simulink model "independentSISO_2023b_mdl"  (R2023b)
settings: Solver=ode4  StartTime=0  StopTime=6e6  FixedStep=0.1  RelTol=1e-3
undefined symbols (not defined in the file): f_ii, g_ii, P0
settings Model: SimulationMode=accelerator  Creator=mohammadodeh  LastModifiedBy=mohammadodeh

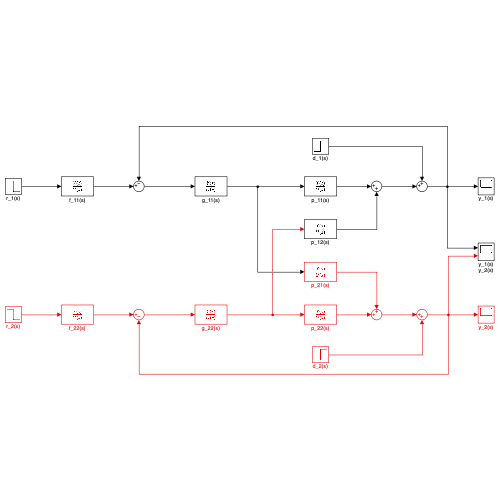
[thumbnail: Simulink's stored preview of the top-level diagram]
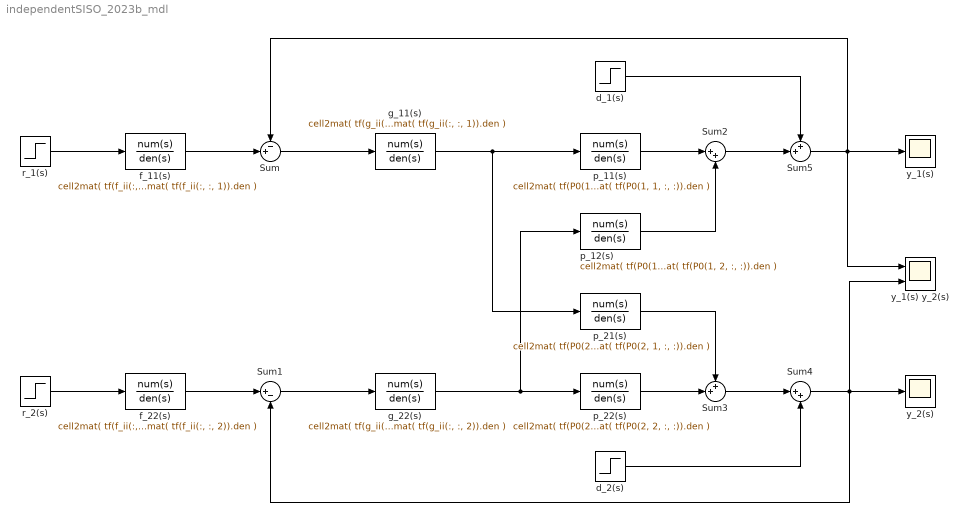
== system independentSISO_2023b_mdl ==
  Sum : Sum  Inputs=-+|
  Sum1 : Sum  Inputs=|+-
  Sum2 : Sum  Inputs=|++
  Sum3 : Sum  Inputs=++|
  Sum4 : Sum  Inputs=|++
  Sum5 : Sum  Inputs=++|
  d_1(s) : Step  Time=4e6  After=0.5  SampleTime=0
  d_2(s) : Step  Time=5e6  After=2  SampleTime=0
  f_11(s) : TransferFcn  Numerator=cell2mat( tf(f_ii(:, :, 1)).num )  Denominator=cell2mat( tf(f_ii(:, :, 1)).den )
  f_22(s) : TransferFcn  Numerator=cell2mat( tf(f_ii(:, :, 2)).num )  Denominator=cell2mat( tf(f_ii(:, :, 2)).den )
  g_11(s) : TransferFcn  Numerator=cell2mat( tf(g_ii(:, :, 1)).num )  Denominator=cell2mat( tf(g_ii(:, :, 1)).den )
  g_22(s) : TransferFcn  Numerator=cell2mat( tf(g_ii(:, :, 2)).num )  Denominator=cell2mat( tf(g_ii(:, :, 2)).den )
  p_11(s) : TransferFcn  Numerator=cell2mat( tf(P0(1, 1, :, :)).num )  Denominator=cell2mat( tf(P0(1, 1, :, :)).den )
  p_12(s) : TransferFcn  Numerator=cell2mat( tf(P0(1, 2, :, :)).num )  Denominator=cell2mat( tf(P0(1, 2, :, :)).den )
  p_21(s) : TransferFcn  Numerator=cell2mat( tf(P0(2, 1, :, :)).num )  Denominator=cell2mat( tf(P0(2, 1, :, :)).den )
  p_22(s) : TransferFcn  Numerator=cell2mat( tf(P0(2, 2, :, :)).num )  Denominator=cell2mat( tf(P0(2, 2, :, :)).den )
  r_1(s) : Step  Time=2e6  Before=2  SampleTime=0
  r_2(s) : Step  Time=3e6  Before=8  After=4  SampleTime=0
  y_1(s) : Scope
  y_1(s) y_2(s) : Scope  NumInputPorts=2
  y_2(s) : Scope
  wires:
  f_11(s)/1 -> Sum/2
  Sum/1 -> g_11(s)/1
  f_22(s)/1 -> Sum1/1
  Sum1/1 -> g_22(s)/1
  g_11(s)/1 -> p_21(s)/1, p_11(s)/1
  g_22(s)/1 -> p_12(s)/1, p_22(s)/1
  r_1(s)/1 -> f_11(s)/1
  r_2(s)/1 -> f_22(s)/1
  Sum4/1 -> y_2(s)/1, Sum1/2, y_1(s) y_2(s)/2
  d_1(s)/1 -> Sum5/1
  Sum5/1 -> y_1(s) y_2(s)/1, Sum/1, y_1(s)/1
  p_21(s)/1 -> Sum3/1
  p_12(s)/1 -> Sum2/2
  d_2(s)/1 -> Sum4/2
  p_22(s)/1 -> Sum3/2
  Sum3/1 -> Sum4/1
  p_11(s)/1 -> Sum2/1
  Sum2/1 -> Sum5/2
